simulink model "LongBoi_String2_Diode"  (R2023b)
settings: Solver=VariableStepAuto  StartTime=0.0  StopTime=1  FixedStep=Ts_Power  MinStep=0.0025  RelTol=1e-4
PreLoadFcn:
  | Ts_Power=5e-4;
  | Slope_Vdc=1;
InitFcn:
  | Ts_Power=50e-6;
  | Tc=1e-5;%break algebraic loop time constant
StopFcn:
  | if exist('I','var') && exist('V','var')
  |    figure(1)
  |    clf
  |    n=find(I>=0);
  |    n=n(end);
  |    Vglobal=V(1:n);
  |    Iglobal=I(1:n);
  | 
  | 
  |    Pglobal=Vglobal.*Iglobal;
  |    n=find(Pglobal==max(Pglobal));
  |    Pmax=Pglobal(n);
  |    Vmp=Vglobal(n);
  |    Imp=Iglobal(n);
  | 
  | 
  |    subplot(211)
  |    plot(Vglobal, Iglobal,Vmp,Imp,'or')
  |    ylabel('Current (A)')
  |    title(sprintf('Global I-V & P-V characteristics\n %s' ,ModuleName))
  | 
  | 
  |    subplot(212)
  |    plot(Vglobal, Pglobal,Vmp,Pmax,'or')
  |    ylabel('Power (W)')
  |    xlabel('Voltage (V)')
  | end
model workspace (MAT data in the model file):
  slope_Vdc = 3.0848387096
values from neighbouring files (symbols this model uses):
  Slope_Vdc_string1 = Slope_Vdc_string(1)    [totPower.m]
libraries: spsPVArrayLib x180, spsVariableResistorLib x180, spsDiodeLib x27, spsCurrentMeasurementLib x1, spsVoltageMeasurementLib x1, spsControlledVoltageSourceLib x1, simulink x1, spspowerguiLib x1
(part 5 of 9)

== system LongBoi_String2_Diode/Subsystem44 ==
  Irr : Inport
  Irr1 : Inport  Port=2
  Irr2 : Inport  Port=3
  Irr3 : Inport  Port=4
  Irr4 : Inport  Port=5
  Irr5 : Inport  Port=6
  Irr6 : Inport  Port=7
  PV1 : Subsystem
      settings: PortSchema="{\"entries\":[{\"content\":{\"sides\":[{\"content\":{\"connectorIds\":[\"In1\"]},\"type\":\"ConnectorPlacement.EquallySpacedRectSide\",\"uuid\":\"5c508248-bd07-48d5-951d-be180bcc8740\"},{\"content\":{\"connectorIds\":[],\"side\":\"RIGHT\"},\"type\":\"ConnectorPlacement.EquallySpacedRectSide\",\"uuid\":\"e31a9bdc-b533-497f-8610-a92a4eef02bc\"},{\"content\":{\"connectorIds\":[\"LConn1\"],\"side\":\"TOP\"},\"type\":\"ConnectorPlacement.EquallySpacedRectSide\",\"uuid\":\"a80efd6c-0c74-41ec-a161-3d709011a457\"},{\"content\":{\"connectorIds\":[\"RConn1\"],\"side\":\"BOTTOM\"},\"type\":\"ConnectorPlacement.EquallySpacedRectSide\",\"uuid\":\"e2d028a7-872a-45fc-84e4-cb840db01281\"}]},\"type\":\"ConnectorPlacement.EquallySpacedConnector\",\"uuid\":\"57d442c0-d58c-4dd4-aeba-72d113e063d7\"}],\"packageUris\":[\"http://schema.mathworks.com/mf0/Connector/19700101\"],\"version\":\"1.0\"}"
  PV2 : Subsystem
      settings: PortSchema="{\"entries\":[{\"content\":{\"sides\":[{\"content\":{\"connectorIds\":[\"In1\"]},\"type\":\"ConnectorPlacement.EquallySpacedRectSide\",\"uuid\":\"5c508248-bd07-48d5-951d-be180bcc8740\"},{\"content\":{\"connectorIds\":[],\"side\":\"RIGHT\"},\"type\":\"ConnectorPlacement.EquallySpacedRectSide\",\"uuid\":\"e31a9bdc-b533-497f-8610-a92a4eef02bc\"},{\"content\":{\"connectorIds\":[\"LConn1\"],\"side\":\"TOP\"},\"type\":\"ConnectorPlacement.EquallySpacedRectSide\",\"uuid\":\"a80efd6c-0c74-41ec-a161-3d709011a457\"},{\"content\":{\"connectorIds\":[\"RConn1\"],\"side\":\"BOTTOM\"},\"type\":\"ConnectorPlacement.EquallySpacedRectSide\",\"uuid\":\"e2d028a7-872a-45fc-84e4-cb840db01281\"}]},\"type\":\"ConnectorPlacement.EquallySpacedConnector\",\"uuid\":\"57d442c0-d58c-4dd4-aeba-72d113e063d7\"}],\"packageUris\":[\"http://schema.mathworks.com/mf0/Connector/19700101\"],\"version\":\"1.0\"}"
  PV3 : Subsystem
      settings: PortSchema="{\"entries\":[{\"content\":{\"sides\":[{\"content\":{\"connectorIds\":[\"In1\"]},\"type\":\"ConnectorPlacement.EquallySpacedRectSide\",\"uuid\":\"5c508248-bd07-48d5-951d-be180bcc8740\"},{\"content\":{\"connectorIds\":[],\"side\":\"RIGHT\"},\"type\":\"ConnectorPlacement.EquallySpacedRectSide\",\"uuid\":\"e31a9bdc-b533-497f-8610-a92a4eef02bc\"},{\"content\":{\"connectorIds\":[\"LConn1\"],\"side\":\"TOP\"},\"type\":\"ConnectorPlacement.EquallySpacedRectSide\",\"uuid\":\"a80efd6c-0c74-41ec-a161-3d709011a457\"},{\"content\":{\"connectorIds\":[\"RConn1\"],\"side\":\"BOTTOM\"},\"type\":\"ConnectorPlacement.EquallySpacedRectSide\",\"uuid\":\"e2d028a7-872a-45fc-84e4-cb840db01281\"}]},\"type\":\"ConnectorPlacement.EquallySpacedConnector\",\"uuid\":\"57d442c0-d58c-4dd4-aeba-72d113e063d7\"}],\"packageUris\":[\"http://schema.mathworks.com/mf0/Connector/19700101\"],\"version\":\"1.0\"}"
  PV4 : Subsystem
      settings: PortSchema="{\"entries\":[{\"content\":{\"sides\":[{\"content\":{\"connectorIds\":[\"In1\"]},\"type\":\"ConnectorPlacement.EquallySpacedRectSide\",\"uuid\":\"5c508248-bd07-48d5-951d-be180bcc8740\"},{\"content\":{\"connectorIds\":[],\"side\":\"RIGHT\"},\"type\":\"ConnectorPlacement.EquallySpacedRectSide\",\"uuid\":\"e31a9bdc-b533-497f-8610-a92a4eef02bc\"},{\"content\":{\"connectorIds\":[\"LConn1\"],\"side\":\"TOP\"},\"type\":\"ConnectorPlacement.EquallySpacedRectSide\",\"uuid\":\"a80efd6c-0c74-41ec-a161-3d709011a457\"},{\"content\":{\"connectorIds\":[\"RConn1\"],\"side\":\"BOTTOM\"},\"type\":\"ConnectorPlacement.EquallySpacedRectSide\",\"uuid\":\"e2d028a7-872a-45fc-84e4-cb840db01281\"}]},\"type\":\"ConnectorPlacement.EquallySpacedConnector\",\"uuid\":\"57d442c0-d58c-4dd4-aeba-72d113e063d7\"}],\"packageUris\":[\"http://schema.mathworks.com/mf0/Connector/19700101\"],\"version\":\"1.0\"}"
  PV5 : Subsystem
      settings: PortSchema="{\"entries\":[{\"content\":{\"sides\":[{\"content\":{\"connectorIds\":[\"In1\"]},\"type\":\"ConnectorPlacement.EquallySpacedRectSide\",\"uuid\":\"5c508248-bd07-48d5-951d-be180bcc8740\"},{\"content\":{\"connectorIds\":[],\"side\":\"RIGHT\"},\"type\":\"ConnectorPlacement.EquallySpacedRectSide\",\"uuid\":\"e31a9bdc-b533-497f-8610-a92a4eef02bc\"},{\"content\":{\"connectorIds\":[\"LConn1\"],\"side\":\"TOP\"},\"type\":\"ConnectorPlacement.EquallySpacedRectSide\",\"uuid\":\"a80efd6c-0c74-41ec-a161-3d709011a457\"},{\"content\":{\"connectorIds\":[\"RConn1\"],\"side\":\"BOTTOM\"},\"type\":\"ConnectorPlacement.EquallySpacedRectSide\",\"uuid\":\"e2d028a7-872a-45fc-84e4-cb840db01281\"}]},\"type\":\"ConnectorPlacement.EquallySpacedConnector\",\"uuid\":\"57d442c0-d58c-4dd4-aeba-72d113e063d7\"}],\"packageUris\":[\"http://schema.mathworks.com/mf0/Connector/19700101\"],\"version\":\"1.0\"}"
  PV6 : Subsystem
      settings: PortSchema="{\"entries\":[{\"content\":{\"sides\":[{\"content\":{\"connectorIds\":[\"In1\"]},\"type\":\"ConnectorPlacement.EquallySpacedRectSide\",\"uuid\":\"5c508248-bd07-48d5-951d-be180bcc8740\"},{\"content\":{\"connectorIds\":[],\"side\":\"RIGHT\"},\"type\":\"ConnectorPlacement.EquallySpacedRectSide\",\"uuid\":\"e31a9bdc-b533-497f-8610-a92a4eef02bc\"},{\"content\":{\"connectorIds\":[\"LConn1\"],\"side\":\"TOP\"},\"type\":\"ConnectorPlacement.EquallySpacedRectSide\",\"uuid\":\"a80efd6c-0c74-41ec-a161-3d709011a457\"},{\"content\":{\"connectorIds\":[\"RConn1\"],\"side\":\"BOTTOM\"},\"type\":\"ConnectorPlacement.EquallySpacedRectSide\",\"uuid\":\"e2d028a7-872a-45fc-84e4-cb840db01281\"}]},\"type\":\"ConnectorPlacement.EquallySpacedConnector\",\"uuid\":\"57d442c0-d58c-4dd4-aeba-72d113e063d7\"}],\"packageUris\":[\"http://schema.mathworks.com/mf0/Connector/19700101\"],\"version\":\"1.0\"}"
  PV7 : Subsystem
      settings: PortSchema="{\"entries\":[{\"content\":{\"sides\":[{\"content\":{\"connectorIds\":[\"In1\"]},\"type\":\"ConnectorPlacement.EquallySpacedRectSide\",\"uuid\":\"5c508248-bd07-48d5-951d-be180bcc8740\"},{\"content\":{\"connectorIds\":[],\"side\":\"RIGHT\"},\"type\":\"ConnectorPlacement.EquallySpacedRectSide\",\"uuid\":\"e31a9bdc-b533-497f-8610-a92a4eef02bc\"},{\"content\":{\"connectorIds\":[\"LConn1\"],\"side\":\"TOP\"},\"type\":\"ConnectorPlacement.EquallySpacedRectSide\",\"uuid\":\"a80efd6c-0c74-41ec-a161-3d709011a457\"},{\"content\":{\"connectorIds\":[\"RConn1\"],\"side\":\"BOTTOM\"},\"type\":\"ConnectorPlacement.EquallySpacedRectSide\",\"uuid\":\"e2d028a7-872a-45fc-84e4-cb840db01281\"}]},\"type\":\"ConnectorPlacement.EquallySpacedConnector\",\"uuid\":\"57d442c0-d58c-4dd4-aeba-72d113e063d7\"}],\"packageUris\":[\"http://schema.mathworks.com/mf0/Connector/19700101\"],\"version\":\"1.0\"}"
  + : PMIOPort  Side=Left
  - : PMIOPort  Port=2  Side=Right
  wires:
  Irr2/1 -> PV4/1(Irr)
  Irr/1 -> PV6/1(Irr)
  Irr1/1 -> PV5/1(Irr)
  Irr3/1 -> PV3/1(Irr)
  Irr5/1 -> PV1/1(Irr)
  Irr4/1 -> PV2/1(Irr)
  Irr6/1 -> PV7/1(Irr)
  connections:
  PV6/LConn1 -- +/RConn1
  PV4/LConn1 -- PV5/RConn1
  PV6/RConn1 -- PV5/LConn1
  PV3/RConn1 -- PV2/LConn1
  PV2/RConn1 -- PV1/LConn1
  PV4/RConn1 -- PV3/LConn1
  -/RConn1 -- PV7/RConn1
  PV7/LConn1 -- PV1/RConn1

== system LongBoi_String2_Diode/Subsystem45 ==
  Irr : Inport
  Irr1 : Inport  Port=2
  Irr2 : Inport  Port=3
  Irr3 : Inport  Port=4
  Irr4 : Inport  Port=5
  Irr5 : Inport  Port=6
  Irr6 : Inport  Port=7
  PV1 : Subsystem
      settings: PortSchema="{\"entries\":[{\"content\":{\"sides\":[{\"content\":{\"connectorIds\":[\"In1\"]},\"type\":\"ConnectorPlacement.EquallySpacedRectSide\",\"uuid\":\"5c508248-bd07-48d5-951d-be180bcc8740\"},{\"content\":{\"connectorIds\":[],\"side\":\"RIGHT\"},\"type\":\"ConnectorPlacement.EquallySpacedRectSide\",\"uuid\":\"e31a9bdc-b533-497f-8610-a92a4eef02bc\"},{\"content\":{\"connectorIds\":[\"LConn1\"],\"side\":\"TOP\"},\"type\":\"ConnectorPlacement.EquallySpacedRectSide\",\"uuid\":\"a80efd6c-0c74-41ec-a161-3d709011a457\"},{\"content\":{\"connectorIds\":[\"RConn1\"],\"side\":\"BOTTOM\"},\"type\":\"ConnectorPlacement.EquallySpacedRectSide\",\"uuid\":\"e2d028a7-872a-45fc-84e4-cb840db01281\"}]},\"type\":\"ConnectorPlacement.EquallySpacedConnector\",\"uuid\":\"57d442c0-d58c-4dd4-aeba-72d113e063d7\"}],\"packageUris\":[\"http://schema.mathworks.com/mf0/Connector/19700101\"],\"version\":\"1.0\"}"
  PV2 : Subsystem
      settings: PortSchema="{\"entries\":[{\"content\":{\"sides\":[{\"content\":{\"connectorIds\":[\"In1\"]},\"type\":\"ConnectorPlacement.EquallySpacedRectSide\",\"uuid\":\"5c508248-bd07-48d5-951d-be180bcc8740\"},{\"content\":{\"connectorIds\":[],\"side\":\"RIGHT\"},\"type\":\"ConnectorPlacement.EquallySpacedRectSide\",\"uuid\":\"e31a9bdc-b533-497f-8610-a92a4eef02bc\"},{\"content\":{\"connectorIds\":[\"LConn1\"],\"side\":\"TOP\"},\"type\":\"ConnectorPlacement.EquallySpacedRectSide\",\"uuid\":\"a80efd6c-0c74-41ec-a161-3d709011a457\"},{\"content\":{\"connectorIds\":[\"RConn1\"],\"side\":\"BOTTOM\"},\"type\":\"ConnectorPlacement.EquallySpacedRectSide\",\"uuid\":\"e2d028a7-872a-45fc-84e4-cb840db01281\"}]},\"type\":\"ConnectorPlacement.EquallySpacedConnector\",\"uuid\":\"57d442c0-d58c-4dd4-aeba-72d113e063d7\"}],\"packageUris\":[\"http://schema.mathworks.com/mf0/Connector/19700101\"],\"version\":\"1.0\"}"
  PV3 : Subsystem
      settings: PortSchema="{\"entries\":[{\"content\":{\"sides\":[{\"content\":{\"connectorIds\":[\"In1\"]},\"type\":\"ConnectorPlacement.EquallySpacedRectSide\",\"uuid\":\"5c508248-bd07-48d5-951d-be180bcc8740\"},{\"content\":{\"connectorIds\":[],\"side\":\"RIGHT\"},\"type\":\"ConnectorPlacement.EquallySpacedRectSide\",\"uuid\":\"e31a9bdc-b533-497f-8610-a92a4eef02bc\"},{\"content\":{\"connectorIds\":[\"LConn1\"],\"side\":\"TOP\"},\"type\":\"ConnectorPlacement.EquallySpacedRectSide\",\"uuid\":\"a80efd6c-0c74-41ec-a161-3d709011a457\"},{\"content\":{\"connectorIds\":[\"RConn1\"],\"side\":\"BOTTOM\"},\"type\":\"ConnectorPlacement.EquallySpacedRectSide\",\"uuid\":\"e2d028a7-872a-45fc-84e4-cb840db01281\"}]},\"type\":\"ConnectorPlacement.EquallySpacedConnector\",\"uuid\":\"57d442c0-d58c-4dd4-aeba-72d113e063d7\"}],\"packageUris\":[\"http://schema.mathworks.com/mf0/Connector/19700101\"],\"version\":\"1.0\"}"
  PV4 : Subsystem
      settings: PortSchema="{\"entries\":[{\"content\":{\"sides\":[{\"content\":{\"connectorIds\":[\"In1\"]},\"type\":\"ConnectorPlacement.EquallySpacedRectSide\",\"uuid\":\"5c508248-bd07-48d5-951d-be180bcc8740\"},{\"content\":{\"connectorIds\":[],\"side\":\"RIGHT\"},\"type\":\"ConnectorPlacement.EquallySpacedRectSide\",\"uuid\":\"e31a9bdc-b533-497f-8610-a92a4eef02bc\"},{\"content\":{\"connectorIds\":[\"LConn1\"],\"side\":\"TOP\"},\"type\":\"ConnectorPlacement.EquallySpacedRectSide\",\"uuid\":\"a80efd6c-0c74-41ec-a161-3d709011a457\"},{\"content\":{\"connectorIds\":[\"RConn1\"],\"side\":\"BOTTOM\"},\"type\":\"ConnectorPlacement.EquallySpacedRectSide\",\"uuid\":\"e2d028a7-872a-45fc-84e4-cb840db01281\"}]},\"type\":\"ConnectorPlacement.EquallySpacedConnector\",\"uuid\":\"57d442c0-d58c-4dd4-aeba-72d113e063d7\"}],\"packageUris\":[\"http://schema.mathworks.com/mf0/Connector/19700101\"],\"version\":\"1.0\"}"
  PV5 : Subsystem
      settings: PortSchema="{\"entries\":[{\"content\":{\"sides\":[{\"content\":{\"connectorIds\":[\"In1\"]},\"type\":\"ConnectorPlacement.EquallySpacedRectSide\",\"uuid\":\"5c508248-bd07-48d5-951d-be180bcc8740\"},{\"content\":{\"connectorIds\":[],\"side\":\"RIGHT\"},\"type\":\"ConnectorPlacement.EquallySpacedRectSide\",\"uuid\":\"e31a9bdc-b533-497f-8610-a92a4eef02bc\"},{\"content\":{\"connectorIds\":[\"LConn1\"],\"side\":\"TOP\"},\"type\":\"ConnectorPlacement.EquallySpacedRectSide\",\"uuid\":\"a80efd6c-0c74-41ec-a161-3d709011a457\"},{\"content\":{\"connectorIds\":[\"RConn1\"],\"side\":\"BOTTOM\"},\"type\":\"ConnectorPlacement.EquallySpacedRectSide\",\"uuid\":\"e2d028a7-872a-45fc-84e4-cb840db01281\"}]},\"type\":\"ConnectorPlacement.EquallySpacedConnector\",\"uuid\":\"57d442c0-d58c-4dd4-aeba-72d113e063d7\"}],\"packageUris\":[\"http://schema.mathworks.com/mf0/Connector/19700101\"],\"version\":\"1.0\"}"
  PV6 : Subsystem
      settings: PortSchema="{\"entries\":[{\"content\":{\"sides\":[{\"content\":{\"connectorIds\":[\"In1\"]},\"type\":\"ConnectorPlacement.EquallySpacedRectSide\",\"uuid\":\"5c508248-bd07-48d5-951d-be180bcc8740\"},{\"content\":{\"connectorIds\":[],\"side\":\"RIGHT\"},\"type\":\"ConnectorPlacement.EquallySpacedRectSide\",\"uuid\":\"e31a9bdc-b533-497f-8610-a92a4eef02bc\"},{\"content\":{\"connectorIds\":[\"LConn1\"],\"side\":\"TOP\"},\"type\":\"ConnectorPlacement.EquallySpacedRectSide\",\"uuid\":\"a80efd6c-0c74-41ec-a161-3d709011a457\"},{\"content\":{\"connectorIds\":[\"RConn1\"],\"side\":\"BOTTOM\"},\"type\":\"ConnectorPlacement.EquallySpacedRectSide\",\"uuid\":\"e2d028a7-872a-45fc-84e4-cb840db01281\"}]},\"type\":\"ConnectorPlacement.EquallySpacedConnector\",\"uuid\":\"57d442c0-d58c-4dd4-aeba-72d113e063d7\"}],\"packageUris\":[\"http://schema.mathworks.com/mf0/Connector/19700101\"],\"version\":\"1.0\"}"
  PV7 : Subsystem
      settings: PortSchema="{\"entries\":[{\"content\":{\"sides\":[{\"content\":{\"connectorIds\":[\"In1\"]},\"type\":\"ConnectorPlacement.EquallySpacedRectSide\",\"uuid\":\"5c508248-bd07-48d5-951d-be180bcc8740\"},{\"content\":{\"connectorIds\":[],\"side\":\"RIGHT\"},\"type\":\"ConnectorPlacement.EquallySpacedRectSide\",\"uuid\":\"e31a9bdc-b533-497f-8610-a92a4eef02bc\"},{\"content\":{\"connectorIds\":[\"LConn1\"],\"side\":\"TOP\"},\"type\":\"ConnectorPlacement.EquallySpacedRectSide\",\"uuid\":\"a80efd6c-0c74-41ec-a161-3d709011a457\"},{\"content\":{\"connectorIds\":[\"RConn1\"],\"side\":\"BOTTOM\"},\"type\":\"ConnectorPlacement.EquallySpacedRectSide\",\"uuid\":\"e2d028a7-872a-45fc-84e4-cb840db01281\"}]},\"type\":\"ConnectorPlacement.EquallySpacedConnector\",\"uuid\":\"57d442c0-d58c-4dd4-aeba-72d113e063d7\"}],\"packageUris\":[\"http://schema.mathworks.com/mf0/Connector/19700101\"],\"version\":\"1.0\"}"
  + : PMIOPort  Side=Left
  - : PMIOPort  Port=2  Side=Right
  wires:
  Irr2/1 -> PV4/1(Irr)
  Irr/1 -> PV6/1(Irr)
  Irr1/1 -> PV5/1(Irr)
  Irr3/1 -> PV3/1(Irr)
  Irr5/1 -> PV1/1(Irr)
  Irr4/1 -> PV2/1(Irr)
  Irr6/1 -> PV7/1(Irr)
  connections:
  PV6/LConn1 -- +/RConn1
  PV4/LConn1 -- PV5/RConn1
  PV6/RConn1 -- PV5/LConn1
  PV3/RConn1 -- PV2/LConn1
  PV2/RConn1 -- PV1/LConn1
  PV4/RConn1 -- PV3/LConn1
  -/RConn1 -- PV7/RConn1
  PV7/LConn1 -- PV1/RConn1

== system LongBoi_String2_Diode/Subsystem55 ==
  Irr : Inport
  Irr1 : Inport  Port=2
  Irr2 : Inport  Port=3
  Irr3 : Inport  Port=4
  Irr4 : Inport  Port=5
  Irr5 : Inport  Port=6
  Irr6 : Inport  Port=7
  PV1 : Subsystem
      settings: PortSchema="{\"entries\":[{\"content\":{\"sides\":[{\"content\":{\"connectorIds\":[\"In1\"]},\"type\":\"ConnectorPlacement.EquallySpacedRectSide\",\"uuid\":\"5c508248-bd07-48d5-951d-be180bcc8740\"},{\"content\":{\"connectorIds\":[],\"side\":\"RIGHT\"},\"type\":\"ConnectorPlacement.EquallySpacedRectSide\",\"uuid\":\"e31a9bdc-b533-497f-8610-a92a4eef02bc\"},{\"content\":{\"connectorIds\":[\"LConn1\"],\"side\":\"TOP\"},\"type\":\"ConnectorPlacement.EquallySpacedRectSide\",\"uuid\":\"a80efd6c-0c74-41ec-a161-3d709011a457\"},{\"content\":{\"connectorIds\":[\"RConn1\"],\"side\":\"BOTTOM\"},\"type\":\"ConnectorPlacement.EquallySpacedRectSide\",\"uuid\":\"e2d028a7-872a-45fc-84e4-cb840db01281\"}]},\"type\":\"ConnectorPlacement.EquallySpacedConnector\",\"uuid\":\"57d442c0-d58c-4dd4-aeba-72d113e063d7\"}],\"packageUris\":[\"http://schema.mathworks.com/mf0/Connector/19700101\"],\"version\":\"1.0\"}"
  PV2 : Subsystem
      settings: PortSchema="{\"entries\":[{\"content\":{\"sides\":[{\"content\":{\"connectorIds\":[\"In1\"]},\"type\":\"ConnectorPlacement.EquallySpacedRectSide\",\"uuid\":\"5c508248-bd07-48d5-951d-be180bcc8740\"},{\"content\":{\"connectorIds\":[],\"side\":\"RIGHT\"},\"type\":\"ConnectorPlacement.EquallySpacedRectSide\",\"uuid\":\"e31a9bdc-b533-497f-8610-a92a4eef02bc\"},{\"content\":{\"connectorIds\":[\"LConn1\"],\"side\":\"TOP\"},\"type\":\"ConnectorPlacement.EquallySpacedRectSide\",\"uuid\":\"a80efd6c-0c74-41ec-a161-3d709011a457\"},{\"content\":{\"connectorIds\":[\"RConn1\"],\"side\":\"BOTTOM\"},\"type\":\"ConnectorPlacement.EquallySpacedRectSide\",\"uuid\":\"e2d028a7-872a-45fc-84e4-cb840db01281\"}]},\"type\":\"ConnectorPlacement.EquallySpacedConnector\",\"uuid\":\"57d442c0-d58c-4dd4-aeba-72d113e063d7\"}],\"packageUris\":[\"http://schema.mathworks.com/mf0/Connector/19700101\"],\"version\":\"1.0\"}"
  PV3 : Subsystem
      settings: PortSchema="{\"entries\":[{\"content\":{\"sides\":[{\"content\":{\"connectorIds\":[\"In1\"]},\"type\":\"ConnectorPlacement.EquallySpacedRectSide\",\"uuid\":\"5c508248-bd07-48d5-951d-be180bcc8740\"},{\"content\":{\"connectorIds\":[],\"side\":\"RIGHT\"},\"type\":\"ConnectorPlacement.EquallySpacedRectSide\",\"uuid\":\"e31a9bdc-b533-497f-8610-a92a4eef02bc\"},{\"content\":{\"connectorIds\":[\"LConn1\"],\"side\":\"TOP\"},\"type\":\"ConnectorPlacement.EquallySpacedRectSide\",\"uuid\":\"a80efd6c-0c74-41ec-a161-3d709011a457\"},{\"content\":{\"connectorIds\":[\"RConn1\"],\"side\":\"BOTTOM\"},\"type\":\"ConnectorPlacement.EquallySpacedRectSide\",\"uuid\":\"e2d028a7-872a-45fc-84e4-cb840db01281\"}]},\"type\":\"ConnectorPlacement.EquallySpacedConnector\",\"uuid\":\"57d442c0-d58c-4dd4-aeba-72d113e063d7\"}],\"packageUris\":[\"http://schema.mathworks.com/mf0/Connector/19700101\"],\"version\":\"1.0\"}"
  PV4 : Subsystem
      settings: PortSchema="{\"entries\":[{\"content\":{\"sides\":[{\"content\":{\"connectorIds\":[\"In1\"]},\"type\":\"ConnectorPlacement.EquallySpacedRectSide\",\"uuid\":\"5c508248-bd07-48d5-951d-be180bcc8740\"},{\"content\":{\"connectorIds\":[],\"side\":\"RIGHT\"},\"type\":\"ConnectorPlacement.EquallySpacedRectSide\",\"uuid\":\"e31a9bdc-b533-497f-8610-a92a4eef02bc\"},{\"content\":{\"connectorIds\":[\"LConn1\"],\"side\":\"TOP\"},\"type\":\"ConnectorPlacement.EquallySpacedRectSide\",\"uuid\":\"a80efd6c-0c74-41ec-a161-3d709011a457\"},{\"content\":{\"connectorIds\":[\"RConn1\"],\"side\":\"BOTTOM\"},\"type\":\"ConnectorPlacement.EquallySpacedRectSide\",\"uuid\":\"e2d028a7-872a-45fc-84e4-cb840db01281\"}]},\"type\":\"ConnectorPlacement.EquallySpacedConnector\",\"uuid\":\"57d442c0-d58c-4dd4-aeba-72d113e063d7\"}],\"packageUris\":[\"http://schema.mathworks.com/mf0/Connector/19700101\"],\"version\":\"1.0\"}"
  PV5 : Subsystem
      settings: PortSchema="{\"entries\":[{\"content\":{\"sides\":[{\"content\":{\"connectorIds\":[\"In1\"]},\"type\":\"ConnectorPlacement.EquallySpacedRectSide\",\"uuid\":\"5c508248-bd07-48d5-951d-be180bcc8740\"},{\"content\":{\"connectorIds\":[],\"side\":\"RIGHT\"},\"type\":\"ConnectorPlacement.EquallySpacedRectSide\",\"uuid\":\"e31a9bdc-b533-497f-8610-a92a4eef02bc\"},{\"content\":{\"connectorIds\":[\"LConn1\"],\"side\":\"TOP\"},\"type\":\"ConnectorPlacement.EquallySpacedRectSide\",\"uuid\":\"a80efd6c-0c74-41ec-a161-3d709011a457\"},{\"content\":{\"connectorIds\":[\"RConn1\"],\"side\":\"BOTTOM\"},\"type\":\"ConnectorPlacement.EquallySpacedRectSide\",\"uuid\":\"e2d028a7-872a-45fc-84e4-cb840db01281\"}]},\"type\":\"ConnectorPlacement.EquallySpacedConnector\",\"uuid\":\"57d442c0-d58c-4dd4-aeba-72d113e063d7\"}],\"packageUris\":[\"http://schema.mathworks.com/mf0/Connector/19700101\"],\"version\":\"1.0\"}"
  PV6 : Subsystem
      settings: PortSchema="{\"entries\":[{\"content\":{\"sides\":[{\"content\":{\"connectorIds\":[\"In1\"]},\"type\":\"ConnectorPlacement.EquallySpacedRectSide\",\"uuid\":\"5c508248-bd07-48d5-951d-be180bcc8740\"},{\"content\":{\"connectorIds\":[],\"side\":\"RIGHT\"},\"type\":\"ConnectorPlacement.EquallySpacedRectSide\",\"uuid\":\"e31a9bdc-b533-497f-8610-a92a4eef02bc\"},{\"content\":{\"connectorIds\":[\"LConn1\"],\"side\":\"TOP\"},\"type\":\"ConnectorPlacement.EquallySpacedRectSide\",\"uuid\":\"a80efd6c-0c74-41ec-a161-3d709011a457\"},{\"content\":{\"connectorIds\":[\"RConn1\"],\"side\":\"BOTTOM\"},\"type\":\"ConnectorPlacement.EquallySpacedRectSide\",\"uuid\":\"e2d028a7-872a-45fc-84e4-cb840db01281\"}]},\"type\":\"ConnectorPlacement.EquallySpacedConnector\",\"uuid\":\"57d442c0-d58c-4dd4-aeba-72d113e063d7\"}],\"packageUris\":[\"http://schema.mathworks.com/mf0/Connector/19700101\"],\"version\":\"1.0\"}"
  PV7 : Subsystem
      settings: PortSchema="{\"entries\":[{\"content\":{\"sides\":[{\"content\":{\"connectorIds\":[\"In1\"]},\"type\":\"ConnectorPlacement.EquallySpacedRectSide\",\"uuid\":\"5c508248-bd07-48d5-951d-be180bcc8740\"},{\"content\":{\"connectorIds\":[],\"side\":\"RIGHT\"},\"type\":\"ConnectorPlacement.EquallySpacedRectSide\",\"uuid\":\"e31a9bdc-b533-497f-8610-a92a4eef02bc\"},{\"content\":{\"connectorIds\":[\"LConn1\"],\"side\":\"TOP\"},\"type\":\"ConnectorPlacement.EquallySpacedRectSide\",\"uuid\":\"a80efd6c-0c74-41ec-a161-3d709011a457\"},{\"content\":{\"connectorIds\":[\"RConn1\"],\"side\":\"BOTTOM\"},\"type\":\"ConnectorPlacement.EquallySpacedRectSide\",\"uuid\":\"e2d028a7-872a-45fc-84e4-cb840db01281\"}]},\"type\":\"ConnectorPlacement.EquallySpacedConnector\",\"uuid\":\"57d442c0-d58c-4dd4-aeba-72d113e063d7\"}],\"packageUris\":[\"http://schema.mathworks.com/mf0/Connector/19700101\"],\"version\":\"1.0\"}"
  + : PMIOPort  Side=Left
  - : PMIOPort  Port=2  Side=Right
  wires:
  Irr2/1 -> PV4/1(Irr)
  Irr/1 -> PV6/1(Irr)
  Irr1/1 -> PV5/1(Irr)
  Irr3/1 -> PV3/1(Irr)
  Irr5/1 -> PV1/1(Irr)
  Irr4/1 -> PV2/1(Irr)
  Irr6/1 -> PV7/1(Irr)
  connections:
  PV6/LConn1 -- +/RConn1
  PV4/LConn1 -- PV5/RConn1
  PV6/RConn1 -- PV5/LConn1
  PV3/RConn1 -- PV2/LConn1
  PV2/RConn1 -- PV1/LConn1
  PV4/RConn1 -- PV3/LConn1
  -/RConn1 -- PV7/RConn1
  PV7/LConn1 -- PV1/RConn1

== system LongBoi_String2_Diode/Subsystem56 ==
  Irr : Inport
  Irr1 : Inport  Port=2
  Irr2 : Inport  Port=3
  Irr3 : Inport  Port=4
  Irr4 : Inport  Port=5
  Irr5 : Inport  Port=6
  Irr6 : Inport  Port=7
  PV1 : Subsystem
      settings: PortSchema="{\"entries\":[{\"content\":{\"sides\":[{\"content\":{\"connectorIds\":[\"In1\"]},\"type\":\"ConnectorPlacement.EquallySpacedRectSide\",\"uuid\":\"5c508248-bd07-48d5-951d-be180bcc8740\"},{\"content\":{\"connectorIds\":[],\"side\":\"RIGHT\"},\"type\":\"ConnectorPlacement.EquallySpacedRectSide\",\"uuid\":\"e31a9bdc-b533-497f-8610-a92a4eef02bc\"},{\"content\":{\"connectorIds\":[\"LConn1\"],\"side\":\"TOP\"},\"type\":\"ConnectorPlacement.EquallySpacedRectSide\",\"uuid\":\"a80efd6c-0c74-41ec-a161-3d709011a457\"},{\"content\":{\"connectorIds\":[\"RConn1\"],\"side\":\"BOTTOM\"},\"type\":\"ConnectorPlacement.EquallySpacedRectSide\",\"uuid\":\"e2d028a7-872a-45fc-84e4-cb840db01281\"}]},\"type\":\"ConnectorPlacement.EquallySpacedConnector\",\"uuid\":\"57d442c0-d58c-4dd4-aeba-72d113e063d7\"}],\"packageUris\":[\"http://schema.mathworks.com/mf0/Connector/19700101\"],\"version\":\"1.0\"}"
  PV2 : Subsystem
      settings: PortSchema="{\"entries\":[{\"content\":{\"sides\":[{\"content\":{\"connectorIds\":[\"In1\"]},\"type\":\"ConnectorPlacement.EquallySpacedRectSide\",\"uuid\":\"5c508248-bd07-48d5-951d-be180bcc8740\"},{\"content\":{\"connectorIds\":[],\"side\":\"RIGHT\"},\"type\":\"ConnectorPlacement.EquallySpacedRectSide\",\"uuid\":\"e31a9bdc-b533-497f-8610-a92a4eef02bc\"},{\"content\":{\"connectorIds\":[\"LConn1\"],\"side\":\"TOP\"},\"type\":\"ConnectorPlacement.EquallySpacedRectSide\",\"uuid\":\"a80efd6c-0c74-41ec-a161-3d709011a457\"},{\"content\":{\"connectorIds\":[\"RConn1\"],\"side\":\"BOTTOM\"},\"type\":\"ConnectorPlacement.EquallySpacedRectSide\",\"uuid\":\"e2d028a7-872a-45fc-84e4-cb840db01281\"}]},\"type\":\"ConnectorPlacement.EquallySpacedConnector\",\"uuid\":\"57d442c0-d58c-4dd4-aeba-72d113e063d7\"}],\"packageUris\":[\"http://schema.mathworks.com/mf0/Connector/19700101\"],\"version\":\"1.0\"}"
  PV3 : Subsystem
      settings: PortSchema="{\"entries\":[{\"content\":{\"sides\":[{\"content\":{\"connectorIds\":[\"In1\"]},\"type\":\"ConnectorPlacement.EquallySpacedRectSide\",\"uuid\":\"5c508248-bd07-48d5-951d-be180bcc8740\"},{\"content\":{\"connectorIds\":[],\"side\":\"RIGHT\"},\"type\":\"ConnectorPlacement.EquallySpacedRectSide\",\"uuid\":\"e31a9bdc-b533-497f-8610-a92a4eef02bc\"},{\"content\":{\"connectorIds\":[\"LConn1\"],\"side\":\"TOP\"},\"type\":\"ConnectorPlacement.EquallySpacedRectSide\",\"uuid\":\"a80efd6c-0c74-41ec-a161-3d709011a457\"},{\"content\":{\"connectorIds\":[\"RConn1\"],\"side\":\"BOTTOM\"},\"type\":\"ConnectorPlacement.EquallySpacedRectSide\",\"uuid\":\"e2d028a7-872a-45fc-84e4-cb840db01281\"}]},\"type\":\"ConnectorPlacement.EquallySpacedConnector\",\"uuid\":\"57d442c0-d58c-4dd4-aeba-72d113e063d7\"}],\"packageUris\":[\"http://schema.mathworks.com/mf0/Connector/19700101\"],\"version\":\"1.0\"}"
  PV4 : Subsystem
      settings: PortSchema="{\"entries\":[{\"content\":{\"sides\":[{\"content\":{\"connectorIds\":[\"In1\"]},\"type\":\"ConnectorPlacement.EquallySpacedRectSide\",\"uuid\":\"5c508248-bd07-48d5-951d-be180bcc8740\"},{\"content\":{\"connectorIds\":[],\"side\":\"RIGHT\"},\"type\":\"ConnectorPlacement.EquallySpacedRectSide\",\"uuid\":\"e31a9bdc-b533-497f-8610-a92a4eef02bc\"},{\"content\":{\"connectorIds\":[\"LConn1\"],\"side\":\"TOP\"},\"type\":\"ConnectorPlacement.EquallySpacedRectSide\",\"uuid\":\"a80efd6c-0c74-41ec-a161-3d709011a457\"},{\"content\":{\"connectorIds\":[\"RConn1\"],\"side\":\"BOTTOM\"},\"type\":\"ConnectorPlacement.EquallySpacedRectSide\",\"uuid\":\"e2d028a7-872a-45fc-84e4-cb840db01281\"}]},\"type\":\"ConnectorPlacement.EquallySpacedConnector\",\"uuid\":\"57d442c0-d58c-4dd4-aeba-72d113e063d7\"}],\"packageUris\":[\"http://schema.mathworks.com/mf0/Connector/19700101\"],\"version\":\"1.0\"}"
  PV5 : Subsystem
      settings: PortSchema="{\"entries\":[{\"content\":{\"sides\":[{\"content\":{\"connectorIds\":[\"In1\"]},\"type\":\"ConnectorPlacement.EquallySpacedRectSide\",\"uuid\":\"5c508248-bd07-48d5-951d-be180bcc8740\"},{\"content\":{\"connectorIds\":[],\"side\":\"RIGHT\"},\"type\":\"ConnectorPlacement.EquallySpacedRectSide\",\"uuid\":\"e31a9bdc-b533-497f-8610-a92a4eef02bc\"},{\"content\":{\"connectorIds\":[\"LConn1\"],\"side\":\"TOP\"},\"type\":\"ConnectorPlacement.EquallySpacedRectSide\",\"uuid\":\"a80efd6c-0c74-41ec-a161-3d709011a457\"},{\"content\":{\"connectorIds\":[\"RConn1\"],\"side\":\"BOTTOM\"},\"type\":\"ConnectorPlacement.EquallySpacedRectSide\",\"uuid\":\"e2d028a7-872a-45fc-84e4-cb840db01281\"}]},\"type\":\"ConnectorPlacement.EquallySpacedConnector\",\"uuid\":\"57d442c0-d58c-4dd4-aeba-72d113e063d7\"}],\"packageUris\":[\"http://schema.mathworks.com/mf0/Connector/19700101\"],\"version\":\"1.0\"}"
  PV6 : Subsystem
      settings: PortSchema="{\"entries\":[{\"content\":{\"sides\":[{\"content\":{\"connectorIds\":[\"In1\"]},\"type\":\"ConnectorPlacement.EquallySpacedRectSide\",\"uuid\":\"5c508248-bd07-48d5-951d-be180bcc8740\"},{\"content\":{\"connectorIds\":[],\"side\":\"RIGHT\"},\"type\":\"ConnectorPlacement.EquallySpacedRectSide\",\"uuid\":\"e31a9bdc-b533-497f-8610-a92a4eef02bc\"},{\"content\":{\"connectorIds\":[\"LConn1\"],\"side\":\"TOP\"},\"type\":\"ConnectorPlacement.EquallySpacedRectSide\",\"uuid\":\"a80efd6c-0c74-41ec-a161-3d709011a457\"},{\"content\":{\"connectorIds\":[\"RConn1\"],\"side\":\"BOTTOM\"},\"type\":\"ConnectorPlacement.EquallySpacedRectSide\",\"uuid\":\"e2d028a7-872a-45fc-84e4-cb840db01281\"}]},\"type\":\"ConnectorPlacement.EquallySpacedConnector\",\"uuid\":\"57d442c0-d58c-4dd4-aeba-72d113e063d7\"}],\"packageUris\":[\"http://schema.mathworks.com/mf0/Connector/19700101\"],\"version\":\"1.0\"}"
  PV7 : Subsystem
      settings: PortSchema="{\"entries\":[{\"content\":{\"sides\":[{\"content\":{\"connectorIds\":[\"In1\"]},\"type\":\"ConnectorPlacement.EquallySpacedRectSide\",\"uuid\":\"5c508248-bd07-48d5-951d-be180bcc8740\"},{\"content\":{\"connectorIds\":[],\"side\":\"RIGHT\"},\"type\":\"ConnectorPlacement.EquallySpacedRectSide\",\"uuid\":\"e31a9bdc-b533-497f-8610-a92a4eef02bc\"},{\"content\":{\"connectorIds\":[\"LConn1\"],\"side\":\"TOP\"},\"type\":\"ConnectorPlacement.EquallySpacedRectSide\",\"uuid\":\"a80efd6c-0c74-41ec-a161-3d709011a457\"},{\"content\":{\"connectorIds\":[\"RConn1\"],\"side\":\"BOTTOM\"},\"type\":\"ConnectorPlacement.EquallySpacedRectSide\",\"uuid\":\"e2d028a7-872a-45fc-84e4-cb840db01281\"}]},\"type\":\"ConnectorPlacement.EquallySpacedConnector\",\"uuid\":\"57d442c0-d58c-4dd4-aeba-72d113e063d7\"}],\"packageUris\":[\"http://schema.mathworks.com/mf0/Connector/19700101\"],\"version\":\"1.0\"}"
  + : PMIOPort  Side=Left
  - : PMIOPort  Port=2  Side=Right
  wires:
  Irr2/1 -> PV4/1(Irr)
  Irr/1 -> PV6/1(Irr)
  Irr1/1 -> PV5/1(Irr)
  Irr3/1 -> PV3/1(Irr)
  Irr5/1 -> PV1/1(Irr)
  Irr4/1 -> PV2/1(Irr)
  Irr6/1 -> PV7/1(Irr)
  connections:
  PV6/LConn1 -- +/RConn1
  PV4/LConn1 -- PV5/RConn1
  PV6/RConn1 -- PV5/LConn1
  PV3/RConn1 -- PV2/LConn1
  PV2/RConn1 -- PV1/LConn1
  PV4/RConn1 -- PV3/LConn1
  -/RConn1 -- PV7/RConn1
  PV7/LConn1 -- PV1/RConn1

== system LongBoi_String2_Diode/Subsystem57 ==
  Irr : Inport
  Irr1 : Inport  Port=2
  Irr2 : Inport  Port=3
  Irr3 : Inport  Port=4
  Irr4 : Inport  Port=5
  Irr5 : Inport  Port=6
  Irr6 : Inport  Port=7
  PV1 : Subsystem
      settings: PortSchema="{\"entries\":[{\"content\":{\"sides\":[{\"content\":{\"connectorIds\":[\"In1\"]},\"type\":\"ConnectorPlacement.EquallySpacedRectSide\",\"uuid\":\"5c508248-bd07-48d5-951d-be180bcc8740\"},{\"content\":{\"connectorIds\":[],\"side\":\"RIGHT\"},\"type\":\"ConnectorPlacement.EquallySpacedRectSide\",\"uuid\":\"e31a9bdc-b533-497f-8610-a92a4eef02bc\"},{\"content\":{\"connectorIds\":[\"LConn1\"],\"side\":\"TOP\"},\"type\":\"ConnectorPlacement.EquallySpacedRectSide\",\"uuid\":\"a80efd6c-0c74-41ec-a161-3d709011a457\"},{\"content\":{\"connectorIds\":[\"RConn1\"],\"side\":\"BOTTOM\"},\"type\":\"ConnectorPlacement.EquallySpacedRectSide\",\"uuid\":\"e2d028a7-872a-45fc-84e4-cb840db01281\"}]},\"type\":\"ConnectorPlacement.EquallySpacedConnector\",\"uuid\":\"57d442c0-d58c-4dd4-aeba-72d113e063d7\"}],\"packageUris\":[\"http://schema.mathworks.com/mf0/Connector/19700101\"],\"version\":\"1.0\"}"
  PV2 : Subsystem
      settings: PortSchema="{\"entries\":[{\"content\":{\"sides\":[{\"content\":{\"connectorIds\":[\"In1\"]},\"type\":\"ConnectorPlacement.EquallySpacedRectSide\",\"uuid\":\"5c508248-bd07-48d5-951d-be180bcc8740\"},{\"content\":{\"connectorIds\":[],\"side\":\"RIGHT\"},\"type\":\"ConnectorPlacement.EquallySpacedRectSide\",\"uuid\":\"e31a9bdc-b533-497f-8610-a92a4eef02bc\"},{\"content\":{\"connectorIds\":[\"LConn1\"],\"side\":\"TOP\"},\"type\":\"ConnectorPlacement.EquallySpacedRectSide\",\"uuid\":\"a80efd6c-0c74-41ec-a161-3d709011a457\"},{\"content\":{\"connectorIds\":[\"RConn1\"],\"side\":\"BOTTOM\"},\"type\":\"ConnectorPlacement.EquallySpacedRectSide\",\"uuid\":\"e2d028a7-872a-45fc-84e4-cb840db01281\"}]},\"type\":\"ConnectorPlacement.EquallySpacedConnector\",\"uuid\":\"57d442c0-d58c-4dd4-aeba-72d113e063d7\"}],\"packageUris\":[\"http://schema.mathworks.com/mf0/Connector/19700101\"],\"version\":\"1.0\"}"
  PV3 : Subsystem
      settings: PortSchema="{\"entries\":[{\"content\":{\"sides\":[{\"content\":{\"connectorIds\":[\"In1\"]},\"type\":\"ConnectorPlacement.EquallySpacedRectSide\",\"uuid\":\"5c508248-bd07-48d5-951d-be180bcc8740\"},{\"content\":{\"connectorIds\":[],\"side\":\"RIGHT\"},\"type\":\"ConnectorPlacement.EquallySpacedRectSide\",\"uuid\":\"e31a9bdc-b533-497f-8610-a92a4eef02bc\"},{\"content\":{\"connectorIds\":[\"LConn1\"],\"side\":\"TOP\"},\"type\":\"ConnectorPlacement.EquallySpacedRectSide\",\"uuid\":\"a80efd6c-0c74-41ec-a161-3d709011a457\"},{\"content\":{\"connectorIds\":[\"RConn1\"],\"side\":\"BOTTOM\"},\"type\":\"ConnectorPlacement.EquallySpacedRectSide\",\"uuid\":\"e2d028a7-872a-45fc-84e4-cb840db01281\"}]},\"type\":\"ConnectorPlacement.EquallySpacedConnector\",\"uuid\":\"57d442c0-d58c-4dd4-aeba-72d113e063d7\"}],\"packageUris\":[\"http://schema.mathworks.com/mf0/Connector/19700101\"],\"version\":\"1.0\"}"
  PV4 : Subsystem
      settings: PortSchema="{\"entries\":[{\"content\":{\"sides\":[{\"content\":{\"connectorIds\":[\"In1\"]},\"type\":\"ConnectorPlacement.EquallySpacedRectSide\",\"uuid\":\"5c508248-bd07-48d5-951d-be180bcc8740\"},{\"content\":{\"connectorIds\":[],\"side\":\"RIGHT\"},\"type\":\"ConnectorPlacement.EquallySpacedRectSide\",\"uuid\":\"e31a9bdc-b533-497f-8610-a92a4eef02bc\"},{\"content\":{\"connectorIds\":[\"LConn1\"],\"side\":\"TOP\"},\"type\":\"ConnectorPlacement.EquallySpacedRectSide\",\"uuid\":\"a80efd6c-0c74-41ec-a161-3d709011a457\"},{\"content\":{\"connectorIds\":[\"RConn1\"],\"side\":\"BOTTOM\"},\"type\":\"ConnectorPlacement.EquallySpacedRectSide\",\"uuid\":\"e2d028a7-872a-45fc-84e4-cb840db01281\"}]},\"type\":\"ConnectorPlacement.EquallySpacedConnector\",\"uuid\":\"57d442c0-d58c-4dd4-aeba-72d113e063d7\"}],\"packageUris\":[\"http://schema.mathworks.com/mf0/Connector/19700101\"],\"version\":\"1.0\"}"
  PV5 : Subsystem
      settings: PortSchema="{\"entries\":[{\"content\":{\"sides\":[{\"content\":{\"connectorIds\":[\"In1\"]},\"type\":\"ConnectorPlacement.EquallySpacedRectSide\",\"uuid\":\"5c508248-bd07-48d5-951d-be180bcc8740\"},{\"content\":{\"connectorIds\":[],\"side\":\"RIGHT\"},\"type\":\"ConnectorPlacement.EquallySpacedRectSide\",\"uuid\":\"e31a9bdc-b533-497f-8610-a92a4eef02bc\"},{\"content\":{\"connectorIds\":[\"LConn1\"],\"side\":\"TOP\"},\"type\":\"ConnectorPlacement.EquallySpacedRectSide\",\"uuid\":\"a80efd6c-0c74-41ec-a161-3d709011a457\"},{\"content\":{\"connectorIds\":[\"RConn1\"],\"side\":\"BOTTOM\"},\"type\":\"ConnectorPlacement.EquallySpacedRectSide\",\"uuid\":\"e2d028a7-872a-45fc-84e4-cb840db01281\"}]},\"type\":\"ConnectorPlacement.EquallySpacedConnector\",\"uuid\":\"57d442c0-d58c-4dd4-aeba-72d113e063d7\"}],\"packageUris\":[\"http://schema.mathworks.com/mf0/Connector/19700101\"],\"version\":\"1.0\"}"
  PV6 : Subsystem
      settings: PortSchema="{\"entries\":[{\"content\":{\"sides\":[{\"content\":{\"connectorIds\":[\"In1\"]},\"type\":\"ConnectorPlacement.EquallySpacedRectSide\",\"uuid\":\"5c508248-bd07-48d5-951d-be180bcc8740\"},{\"content\":{\"connectorIds\":[],\"side\":\"RIGHT\"},\"type\":\"ConnectorPlacement.EquallySpacedRectSide\",\"uuid\":\"e31a9bdc-b533-497f-8610-a92a4eef02bc\"},{\"content\":{\"connectorIds\":[\"LConn1\"],\"side\":\"TOP\"},\"type\":\"ConnectorPlacement.EquallySpacedRectSide\",\"uuid\":\"a80efd6c-0c74-41ec-a161-3d709011a457\"},{\"content\":{\"connectorIds\":[\"RConn1\"],\"side\":\"BOTTOM\"},\"type\":\"ConnectorPlacement.EquallySpacedRectSide\",\"uuid\":\"e2d028a7-872a-45fc-84e4-cb840db01281\"}]},\"type\":\"ConnectorPlacement.EquallySpacedConnector\",\"uuid\":\"57d442c0-d58c-4dd4-aeba-72d113e063d7\"}],\"packageUris\":[\"http://schema.mathworks.com/mf0/Connector/19700101\"],\"version\":\"1.0\"}"
  PV7 : Subsystem
      settings: PortSchema="{\"entries\":[{\"content\":{\"sides\":[{\"content\":{\"connectorIds\":[\"In1\"]},\"type\":\"ConnectorPlacement.EquallySpacedRectSide\",\"uuid\":\"5c508248-bd07-48d5-951d-be180bcc8740\"},{\"content\":{\"connectorIds\":[],\"side\":\"RIGHT\"},\"type\":\"ConnectorPlacement.EquallySpacedRectSide\",\"uuid\":\"e31a9bdc-b533-497f-8610-a92a4eef02bc\"},{\"content\":{\"connectorIds\":[\"LConn1\"],\"side\":\"TOP\"},\"type\":\"ConnectorPlacement.EquallySpacedRectSide\",\"uuid\":\"a80efd6c-0c74-41ec-a161-3d709011a457\"},{\"content\":{\"connectorIds\":[\"RConn1\"],\"side\":\"BOTTOM\"},\"type\":\"ConnectorPlacement.EquallySpacedRectSide\",\"uuid\":\"e2d028a7-872a-45fc-84e4-cb840db01281\"}]},\"type\":\"ConnectorPlacement.EquallySpacedConnector\",\"uuid\":\"57d442c0-d58c-4dd4-aeba-72d113e063d7\"}],\"packageUris\":[\"http://schema.mathworks.com/mf0/Connector/19700101\"],\"version\":\"1.0\"}"
  + : PMIOPort  Side=Left
  - : PMIOPort  Port=2  Side=Right
  wires:
  Irr2/1 -> PV4/1(Irr)
  Irr/1 -> PV6/1(Irr)
  Irr1/1 -> PV5/1(Irr)
  Irr3/1 -> PV3/1(Irr)
  Irr5/1 -> PV1/1(Irr)
  Irr4/1 -> PV2/1(Irr)
  Irr6/1 -> PV7/1(Irr)
  connections:
  PV6/LConn1 -- +/RConn1
  PV4/LConn1 -- PV5/RConn1
  PV6/RConn1 -- PV5/LConn1
  PV3/RConn1 -- PV2/LConn1
  PV2/RConn1 -- PV1/LConn1
  PV4/RConn1 -- PV3/LConn1
  -/RConn1 -- PV7/RConn1
  PV7/LConn1 -- PV1/RConn1

== system LongBoi_String2_Diode/Subsystem58 ==
  Irr : Inport
  Irr1 : Inport  Port=2
  Irr2 : Inport  Port=3
  Irr3 : Inport  Port=4
  Irr4 : Inport  Port=5
  Irr5 : Inport  Port=6
  Irr6 : Inport  Port=7
  PV1 : Subsystem
      settings: PortSchema="{\"entries\":[{\"content\":{\"sides\":[{\"content\":{\"connectorIds\":[\"In1\"]},\"type\":\"ConnectorPlacement.EquallySpacedRectSide\",\"uuid\":\"5c508248-bd07-48d5-951d-be180bcc8740\"},{\"content\":{\"connectorIds\":[],\"side\":\"RIGHT\"},\"type\":\"ConnectorPlacement.EquallySpacedRectSide\",\"uuid\":\"e31a9bdc-b533-497f-8610-a92a4eef02bc\"},{\"content\":{\"connectorIds\":[\"LConn1\"],\"side\":\"TOP\"},\"type\":\"ConnectorPlacement.EquallySpacedRectSide\",\"uuid\":\"a80efd6c-0c74-41ec-a161-3d709011a457\"},{\"content\":{\"connectorIds\":[\"RConn1\"],\"side\":\"BOTTOM\"},\"type\":\"ConnectorPlacement.EquallySpacedRectSide\",\"uuid\":\"e2d028a7-872a-45fc-84e4-cb840db01281\"}]},\"type\":\"ConnectorPlacement.EquallySpacedConnector\",\"uuid\":\"57d442c0-d58c-4dd4-aeba-72d113e063d7\"}],\"packageUris\":[\"http://schema.mathworks.com/mf0/Connector/19700101\"],\"version\":\"1.0\"}"
  PV2 : Subsystem
      settings: PortSchema="{\"entries\":[{\"content\":{\"sides\":[{\"content\":{\"connectorIds\":[\"In1\"]},\"type\":\"ConnectorPlacement.EquallySpacedRectSide\",\"uuid\":\"5c508248-bd07-48d5-951d-be180bcc8740\"},{\"content\":{\"connectorIds\":[],\"side\":\"RIGHT\"},\"type\":\"ConnectorPlacement.EquallySpacedRectSide\",\"uuid\":\"e31a9bdc-b533-497f-8610-a92a4eef02bc\"},{\"content\":{\"connectorIds\":[\"LConn1\"],\"side\":\"TOP\"},\"type\":\"ConnectorPlacement.EquallySpacedRectSide\",\"uuid\":\"a80efd6c-0c74-41ec-a161-3d709011a457\"},{\"content\":{\"connectorIds\":[\"RConn1\"],\"side\":\"BOTTOM\"},\"type\":\"ConnectorPlacement.EquallySpacedRectSide\",\"uuid\":\"e2d028a7-872a-45fc-84e4-cb840db01281\"}]},\"type\":\"ConnectorPlacement.EquallySpacedConnector\",\"uuid\":\"57d442c0-d58c-4dd4-aeba-72d113e063d7\"}],\"packageUris\":[\"http://schema.mathworks.com/mf0/Connector/19700101\"],\"version\":\"1.0\"}"
  PV3 : Subsystem
      settings: PortSchema="{\"entries\":[{\"content\":{\"sides\":[{\"content\":{\"connectorIds\":[\"In1\"]},\"type\":\"ConnectorPlacement.EquallySpacedRectSide\",\"uuid\":\"5c508248-bd07-48d5-951d-be180bcc8740\"},{\"content\":{\"connectorIds\":[],\"side\":\"RIGHT\"},\"type\":\"ConnectorPlacement.EquallySpacedRectSide\",\"uuid\":\"e31a9bdc-b533-497f-8610-a92a4eef02bc\"},{\"content\":{\"connectorIds\":[\"LConn1\"],\"side\":\"TOP\"},\"type\":\"ConnectorPlacement.EquallySpacedRectSide\",\"uuid\":\"a80efd6c-0c74-41ec-a161-3d709011a457\"},{\"content\":{\"connectorIds\":[\"RConn1\"],\"side\":\"BOTTOM\"},\"type\":\"ConnectorPlacement.EquallySpacedRectSide\",\"uuid\":\"e2d028a7-872a-45fc-84e4-cb840db01281\"}]},\"type\":\"ConnectorPlacement.EquallySpacedConnector\",\"uuid\":\"57d442c0-d58c-4dd4-aeba-72d113e063d7\"}],\"packageUris\":[\"http://schema.mathworks.com/mf0/Connector/19700101\"],\"version\":\"1.0\"}"
  PV4 : Subsystem
      settings: PortSchema="{\"entries\":[{\"content\":{\"sides\":[{\"content\":{\"connectorIds\":[\"In1\"]},\"type\":\"ConnectorPlacement.EquallySpacedRectSide\",\"uuid\":\"5c508248-bd07-48d5-951d-be180bcc8740\"},{\"content\":{\"connectorIds\":[],\"side\":\"RIGHT\"},\"type\":\"ConnectorPlacement.EquallySpacedRectSide\",\"uuid\":\"e31a9bdc-b533-497f-8610-a92a4eef02bc\"},{\"content\":{\"connectorIds\":[\"LConn1\"],\"side\":\"TOP\"},\"type\":\"ConnectorPlacement.EquallySpacedRectSide\",\"uuid\":\"a80efd6c-0c74-41ec-a161-3d709011a457\"},{\"content\":{\"connectorIds\":[\"RConn1\"],\"side\":\"BOTTOM\"},\"type\":\"ConnectorPlacement.EquallySpacedRectSide\",\"uuid\":\"e2d028a7-872a-45fc-84e4-cb840db01281\"}]},\"type\":\"ConnectorPlacement.EquallySpacedConnector\",\"uuid\":\"57d442c0-d58c-4dd4-aeba-72d113e063d7\"}],\"packageUris\":[\"http://schema.mathworks.com/mf0/Connector/19700101\"],\"version\":\"1.0\"}"
  PV5 : Subsystem
      settings: PortSchema="{\"entries\":[{\"content\":{\"sides\":[{\"content\":{\"connectorIds\":[\"In1\"]},\"type\":\"ConnectorPlacement.EquallySpacedRectSide\",\"uuid\":\"5c508248-bd07-48d5-951d-be180bcc8740\"},{\"content\":{\"connectorIds\":[],\"side\":\"RIGHT\"},\"type\":\"ConnectorPlacement.EquallySpacedRectSide\",\"uuid\":\"e31a9bdc-b533-497f-8610-a92a4eef02bc\"},{\"content\":{\"connectorIds\":[\"LConn1\"],\"side\":\"TOP\"},\"type\":\"ConnectorPlacement.EquallySpacedRectSide\",\"uuid\":\"a80efd6c-0c74-41ec-a161-3d709011a457\"},{\"content\":{\"connectorIds\":[\"RConn1\"],\"side\":\"BOTTOM\"},\"type\":\"ConnectorPlacement.EquallySpacedRectSide\",\"uuid\":\"e2d028a7-872a-45fc-84e4-cb840db01281\"}]},\"type\":\"ConnectorPlacement.EquallySpacedConnector\",\"uuid\":\"57d442c0-d58c-4dd4-aeba-72d113e063d7\"}],\"packageUris\":[\"http://schema.mathworks.com/mf0/Connector/19700101\"],\"version\":\"1.0\"}"
  PV6 : Subsystem
      settings: PortSchema="{\"entries\":[{\"content\":{\"sides\":[{\"content\":{\"connectorIds\":[\"In1\"]},\"type\":\"ConnectorPlacement.EquallySpacedRectSide\",\"uuid\":\"5c508248-bd07-48d5-951d-be180bcc8740\"},{\"content\":{\"connectorIds\":[],\"side\":\"RIGHT\"},\"type\":\"ConnectorPlacement.EquallySpacedRectSide\",\"uuid\":\"e31a9bdc-b533-497f-8610-a92a4eef02bc\"},{\"content\":{\"connectorIds\":[\"LConn1\"],\"side\":\"TOP\"},\"type\":\"ConnectorPlacement.EquallySpacedRectSide\",\"uuid\":\"a80efd6c-0c74-41ec-a161-3d709011a457\"},{\"content\":{\"connectorIds\":[\"RConn1\"],\"side\":\"BOTTOM\"},\"type\":\"ConnectorPlacement.EquallySpacedRectSide\",\"uuid\":\"e2d028a7-872a-45fc-84e4-cb840db01281\"}]},\"type\":\"ConnectorPlacement.EquallySpacedConnector\",\"uuid\":\"57d442c0-d58c-4dd4-aeba-72d113e063d7\"}],\"packageUris\":[\"http://schema.mathworks.com/mf0/Connector/19700101\"],\"version\":\"1.0\"}"
  PV7 : Subsystem
      settings: PortSchema="{\"entries\":[{\"content\":{\"sides\":[{\"content\":{\"connectorIds\":[\"In1\"]},\"type\":\"ConnectorPlacement.EquallySpacedRectSide\",\"uuid\":\"5c508248-bd07-48d5-951d-be180bcc8740\"},{\"content\":{\"connectorIds\":[],\"side\":\"RIGHT\"},\"type\":\"ConnectorPlacement.EquallySpacedRectSide\",\"uuid\":\"e31a9bdc-b533-497f-8610-a92a4eef02bc\"},{\"content\":{\"connectorIds\":[\"LConn1\"],\"side\":\"TOP\"},\"type\":\"ConnectorPlacement.EquallySpacedRectSide\",\"uuid\":\"a80efd6c-0c74-41ec-a161-3d709011a457\"},{\"content\":{\"connectorIds\":[\"RConn1\"],\"side\":\"BOTTOM\"},\"type\":\"ConnectorPlacement.EquallySpacedRectSide\",\"uuid\":\"e2d028a7-872a-45fc-84e4-cb840db01281\"}]},\"type\":\"ConnectorPlacement.EquallySpacedConnector\",\"uuid\":\"57d442c0-d58c-4dd4-aeba-72d113e063d7\"}],\"packageUris\":[\"http://schema.mathworks.com/mf0/Connector/19700101\"],\"version\":\"1.0\"}"
  + : PMIOPort  Side=Left
  - : PMIOPort  Port=2  Side=Right
  wires:
  Irr2/1 -> PV4/1(Irr)
  Irr/1 -> PV6/1(Irr)
  Irr1/1 -> PV5/1(Irr)
  Irr3/1 -> PV3/1(Irr)
  Irr5/1 -> PV1/1(Irr)
  Irr4/1 -> PV2/1(Irr)
  Irr6/1 -> PV7/1(Irr)
  connections:
  PV6/LConn1 -- +/RConn1
  PV4/LConn1 -- PV5/RConn1
  PV6/RConn1 -- PV5/LConn1
  PV3/RConn1 -- PV2/LConn1
  PV2/RConn1 -- PV1/LConn1
  PV4/RConn1 -- PV3/LConn1
  -/RConn1 -- PV7/RConn1
  PV7/LConn1 -- PV1/RConn1

== system LongBoi_String2_Diode/Variable DC Source1 ==
  Controlled Voltage Source : spsControlledVoltageSourceLib/Controlled Voltage Source  Initialize=on  Source_Type=DC  Amplitude=0  Phase=0  Frequency=0  Measurements=None
  Slope Vdc : simulink/Sources/Ramp  slope=Slope_Vdc_string1  start=0  InitialOutput=0
  + : PMIOPort  Side=Left
  - : PMIOPort  Port=2  Side=Left
  wires:
  Slope Vdc/1 -> Controlled Voltage Source/1
  connections:
  Controlled Voltage Source/LConn1 -- -/RConn1
  +/RConn1 -- Controlled Voltage Source/RConn1

== system LongBoi_String2_Diode/Subsystem17/PV1 ==
  Irr : Inport
  1PΩ : Constant  Value=1e15
  PV2 : spsPVArrayLib/PV Array  Npar=1  Nser=1  PlotType=array @ 25 deg.C & specified irradiances  S_vec="[ 1000  500  100 ]"  Temp_C_vec="[ 45 25  ]"  ModuleName=User-defined  PlotWhenSelected=off  Pm=3.8061  Ncell=1  Voc=0.7315  Isc=6.41  Vm=0.626  Im=6.08  beta_Voc_pc=-0.2256195755  alpha_Isc_pc=0.04692556634  beta_Voc=-0.0016504  alpha_Isc=0.0030079  IL=6.4137  I0=6.5578e-13  nI=0.95237  Rsh=7.312  Rs=0.0042689  RobustModel=on  RobustCellTemperature=25  BAL=on  Tc=1e-5  Tfilter=5e-5
  Terminator1 : Terminator
  Variable Resistor2 : spsVariableResistorLib/Variable Resistor  Rabsmin=1e-3
      settings: LibrarySourceBlock=sps_lib/Passives/Variable Resistor
  + : PMIOPort  Side=Left
  - : PMIOPort  Port=2  Side=Right
  wires:
  Irr/1 -> PV2/1
  1PΩ/1 -> Variable Resistor2/1
  PV2/1 -> Terminator1/1
  connections:
  -/RConn1 -- Variable Resistor2/RConn1 -- PV2/RConn2
  +/RConn1 -- Variable Resistor2/LConn1 -- PV2/RConn1

== system LongBoi_String2_Diode/Subsystem17/PV2 ==
  Irr : Inport
  1PΩ : Constant  Value=1e15
  PV2 : spsPVArrayLib/PV Array  Npar=1  Nser=1  PlotType=array @ 25 deg.C & specified irradiances  S_vec="[ 1000  500  100 ]"  Temp_C_vec="[ 45 25  ]"  ModuleName=User-defined  PlotWhenSelected=off  Pm=3.8061  Ncell=1  Voc=0.7315  Isc=6.41  Vm=0.626  Im=6.08  beta_Voc_pc=-0.2256195755  alpha_Isc_pc=0.04692556634  beta_Voc=-0.0016504  alpha_Isc=0.0030079  IL=6.4137  I0=6.5578e-13  nI=0.95237  Rsh=7.312  Rs=0.0042689  RobustModel=on  RobustCellTemperature=25  BAL=on  Tc=1e-5  Tfilter=5e-5
  Terminator1 : Terminator
  Variable Resistor2 : spsVariableResistorLib/Variable Resistor  Rabsmin=1e-3
      settings: LibrarySourceBlock=sps_lib/Passives/Variable Resistor
  + : PMIOPort  Side=Left
  - : PMIOPort  Port=2  Side=Right
  wires:
  Irr/1 -> PV2/1
  1PΩ/1 -> Variable Resistor2/1
  PV2/1 -> Terminator1/1
  connections:
  -/RConn1 -- Variable Resistor2/RConn1 -- PV2/RConn2
  +/RConn1 -- Variable Resistor2/LConn1 -- PV2/RConn1

== system LongBoi_String2_Diode/Subsystem17/PV3 ==
  Irr : Inport
  1PΩ : Constant  Value=1e15
  PV2 : spsPVArrayLib/PV Array  Npar=1  Nser=1  PlotType=array @ 25 deg.C & specified irradiances  S_vec="[ 1000  500  100 ]"  Temp_C_vec="[ 45 25  ]"  ModuleName=User-defined  PlotWhenSelected=off  Pm=3.8061  Ncell=1  Voc=0.7315  Isc=6.41  Vm=0.626  Im=6.08  beta_Voc_pc=-0.2256195755  alpha_Isc_pc=0.04692556634  beta_Voc=-0.0016504  alpha_Isc=0.0030079  IL=6.4137  I0=6.5578e-13  nI=0.95237  Rsh=7.312  Rs=0.0042689  RobustModel=on  RobustCellTemperature=25  BAL=on  Tc=1e-5  Tfilter=5e-5
  Terminator1 : Terminator
  Variable Resistor2 : spsVariableResistorLib/Variable Resistor  Rabsmin=1e-3
      settings: LibrarySourceBlock=sps_lib/Passives/Variable Resistor
  + : PMIOPort  Side=Left
  - : PMIOPort  Port=2  Side=Right
  wires:
  Irr/1 -> PV2/1
  1PΩ/1 -> Variable Resistor2/1
  PV2/1 -> Terminator1/1
  connections:
  -/RConn1 -- Variable Resistor2/RConn1 -- PV2/RConn2
  +/RConn1 -- Variable Resistor2/LConn1 -- PV2/RConn1

== system LongBoi_String2_Diode/Subsystem17/PV4 ==
  Irr : Inport
  1PΩ : Constant  Value=1e15
  PV2 : spsPVArrayLib/PV Array  Npar=1  Nser=1  PlotType=array @ 25 deg.C & specified irradiances  S_vec="[ 1000  500  100 ]"  Temp_C_vec="[ 45 25  ]"  ModuleName=User-defined  PlotWhenSelected=off  Pm=3.8061  Ncell=1  Voc=0.7315  Isc=6.41  Vm=0.626  Im=6.08  beta_Voc_pc=-0.2256195755  alpha_Isc_pc=0.04692556634  beta_Voc=-0.0016504  alpha_Isc=0.0030079  IL=6.4137  I0=6.5578e-13  nI=0.95237  Rsh=7.312  Rs=0.0042689  RobustModel=on  RobustCellTemperature=25  BAL=on  Tc=1e-5  Tfilter=5e-5
  Terminator1 : Terminator
  Variable Resistor2 : spsVariableResistorLib/Variable Resistor  Rabsmin=1e-3
      settings: LibrarySourceBlock=sps_lib/Passives/Variable Resistor
  + : PMIOPort  Side=Left
  - : PMIOPort  Port=2  Side=Right
  wires:
  Irr/1 -> PV2/1
  1PΩ/1 -> Variable Resistor2/1
  PV2/1 -> Terminator1/1
  connections:
  -/RConn1 -- Variable Resistor2/RConn1 -- PV2/RConn2
  +/RConn1 -- Variable Resistor2/LConn1 -- PV2/RConn1
